simulink model "uz_dutycyclemeas"  (R2024a)
settings: Solver=FixedStepDiscrete  StartTime=0.0  StopTime=0.2e-3  RelTol=1e-3
values from neighbouring files (symbols this model uses):
  t_clk = 1/f_clk    (= 1e-08)    [uz_dutycyclemeas_init.m]
  t_clk_sig = 1/f_clk_sig    (= 0.000108695652174)    [uz_dutycyclemeas_init.m]
libraries: simulink x2, hdlsllib x1
settings Model: DataTypeOverride=Off  Creator=Geiger  LastModifiedBy=Geiger
settings SolverCC: AlgebraicLoopSolver=TrustRegion
settings DataIOCC: LimitDataPoints=on  SaveOutput=off  SaveTime=off
settings OptimizationCC: BlockReduction=off  ConditionallyExecuteInputs=off  DefaultParameterBehavior=Inlined  LifeSpan=inf
settings DebuggingCC: AlgebraicLoopMsg=error  SingleTaskRateTransMsg=error  UnconnectedInputMsg=warning  UnconnectedOutputMsg=warning  UnconnectedLineMsg=warning  AllowSymbolicDim=off  StrictBusMsg=ErrorOnBusTreatedAsVector  SFUnexpectedBacktrackingDiag=warning  SFNoUnconditionalDefaultTransitionDiag=warning  SFExecutionAtInitializationDiag=none  ArithmeticOperatorsInVariantConditions=warning
settings HardwareCC: ProdBitPerPointer=32  ProdBitPerSizeT=32  ProdBitPerPtrDiffT=32  ProdLargestAtomicFloat=None  ProdIntDivRoundTo=Undefined  ProdEndianess=Unspecified  ProdWordSize=32  ProdHWDeviceType=ASIC/FPGA->ASIC/FPGA  ProdEqTarget=off
settings ModelReferenceCC: EnableRefExpFcnMdlSchedulingChecks=on
settings SFSimCC: SimUseLocalCustomCode=off  CustomCodeUndefinedFunction=UseInterfaceOnly
settings RTWCC: RTWUseLocalCustomCode=off  GPUComputeCapability=3.5
settings CodeAppCC: StateflowObjectComments=on
settings GRTTargetCC: TargetLangStandard=C89/C90 (ANSI)
settings ConfigComp: CovScope=ReferencedModels  CovMetricSettings=dw  CovSaveCumulativeToWorkspaceVar=on  CovSaveSingleToWorkspaceVar=on  CovExternalEMLEnable=off  CovSFcnEnable=off

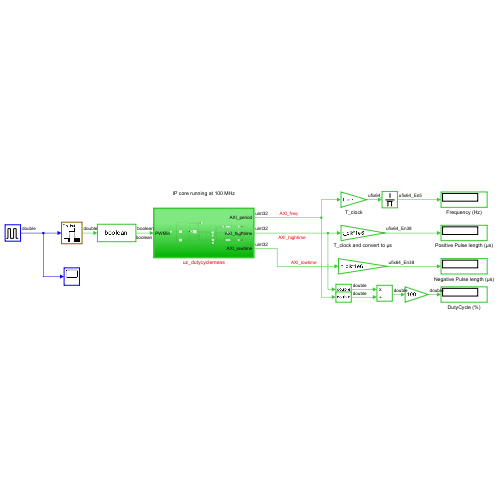
[thumbnail: Simulink's stored preview of the top-level diagram]
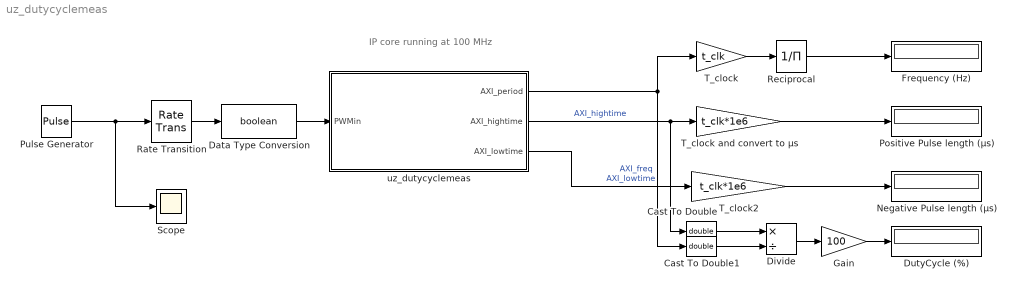
== system uz_dutycyclemeas ==
  note: IP core running at 100 MHz
  Cast To Double : DataTypeConversion  OutDataTypeStr=double  SaturateOnIntegerOverflow=off  RndMeth=Floor
  Cast To Double1 : DataTypeConversion  OutDataTypeStr=double  SaturateOnIntegerOverflow=off  RndMeth=Floor
  Data Type Conversion : DataTypeConversion  OutDataTypeStr=boolean  SaturateOnIntegerOverflow=off  RndMeth=Floor
  Divide : Product  Inputs=*/
  DutyCycle (%) : Display
  Frequency (Hz) : Display
  Gain : Gain  Gain=100
  Negative Pulse length (µs) : Display
  Positive Pulse length (µs) : Display
  Pulse Generator : DiscretePulseGenerator  PulseType=Time based  Period=t_clk_sig  PulseWidth=7.52
  Rate Transition : RateTransition  Deterministic=off  OutPortSampleTime=t_clk
  Reciprocal : Product  Inputs=/
  Scope : Scope
  T_clock : Gain  Gain=t_clk
  T_clock and convert to µs : Gain  Gain=t_clk*1e6
  T_clock2 : Gain  Gain=t_clk*1e6
  uz_dutycyclemeas : Subsystem  TreatAsAtomicUnit=on
  wires:
  uz_dutycyclemeas/2(AXI_hightime) -> Cast To Double/1, T_clock and convert to µs/1  "AXI_hightime"
  Gain/1 -> DutyCycle (%)/1
  uz_dutycyclemeas/3(AXI_lowtime) -> T_clock2/1  "AXI_lowtime"
  Reciprocal/1 -> Frequency (Hz)/1
  T_clock/1 -> Reciprocal/1
  T_clock2/1 -> Negative Pulse length (µs)/1
  uz_dutycyclemeas/1(AXI_period) -> T_clock/1, Cast To Double1/1  "AXI_freq"
  Pulse Generator/1 -> Scope/1, Rate Transition/1
  Data Type Conversion/1 -> uz_dutycyclemeas/1(PWMin)
  Rate Transition/1 -> Data Type Conversion/1
  Divide/1 -> Gain/1
  T_clock and convert to µs/1 -> Positive Pulse length (µs)/1
  Cast To Double/1 -> Divide/1
  Cast To Double1/1 -> Divide/2

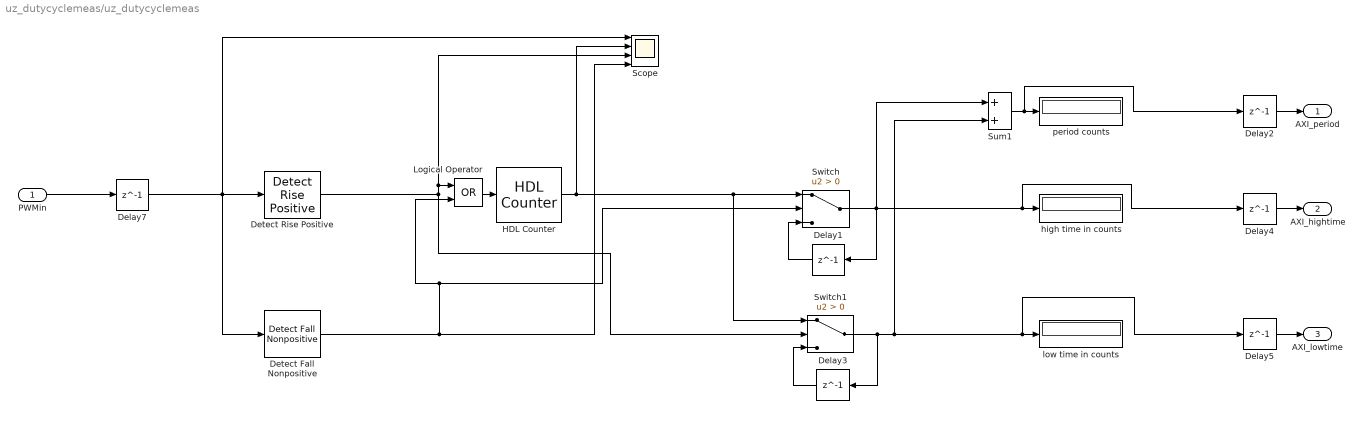
== system uz_dutycyclemeas/uz_dutycyclemeas ==
  PWMin : Inport  OutDataTypeStr=boolean
  Delay{1..5,7} (6 alike) : Delay  DelayLength=1
  Detect Fall Nonpositive : simulink/Logic and Bit Operations/Detect Fall Nonpositive  vinit=0  OutDataTypeStr=boolean
  Detect Rise Positive : simulink/Logic and Bit Operations/Detect Rise Positive  vinit=0  OutDataTypeStr=boolean
  HDL Counter : hdlsllib/Sources/HDL Counter  CountType=Count limited  CountInit=1  CountStep=1  CountMax=2500000  CountFromType=Specify  CountFrom=1  CountResetPort=on  CountLoadPort=off  CountEnbPort=off  CountDirPort=off  CountHitOutputPort=off  CountDataType=Unsigned  CountWordLen=32  CountFracLen=0  CountSampTime=1
  Logical Operator : Logic  Operator=OR  AllPortsSameDT=off  OutDataTypeStr=boolean
  Scope : Scope  NumInputPorts=4
  Sum1 : Sum  AccumDataTypeStr=uint32
  Switch : Switch  Criteria=u2 > Threshold  SaturateOnIntegerOverflow=off  InputSameDT=off
  Switch1 : Switch  Criteria=u2 > Threshold  SaturateOnIntegerOverflow=off  InputSameDT=off
  high time in counts : Display
  low time in counts : Display
  period counts : Display
  AXI_period : Outport  VectorParamsAs1DForOutWhenUnconnected=off
  AXI_hightime : Outport  Port=2  VectorParamsAs1DForOutWhenUnconnected=off
  AXI_lowtime : Outport  Port=3  VectorParamsAs1DForOutWhenUnconnected=off
  wires:
  Switch/1 -> Sum1/1, Delay4/1, high time in counts/1, Delay1/1
  Logical Operator/1 -> HDL Counter/1
  Detect Fall Nonpositive/1 -> Logical Operator/2, Switch/2, Scope/4
  Delay4/1 -> AXI_hightime/1
  Detect Rise Positive/1 -> Switch1/2, Logical Operator/1, Scope/3
  PWMin/1 -> Delay7/1
  Delay5/1 -> AXI_lowtime/1
  Delay2/1 -> AXI_period/1
  Switch1/1 -> Sum1/2, Delay5/1, low time in counts/1, Delay3/1
  Delay1/1 -> Switch/3
  Delay7/1 -> Detect Fall Nonpositive/1, Scope/1, Detect Rise Positive/1
  Delay3/1 -> Switch1/3
  Sum1/1 -> Delay2/1, period counts/1
  HDL Counter/1 -> Switch1/1, Switch/1, Scope/2
